simulink model "atrias_system"  (R2015a)
settings: Solver=FixedStepDiscrete  StartTime=0.0  StopTime=inf  FixedStep=sample_time  RelTol=1e-3
undefined symbols (not defined in the file or in its folder): gui_disable_cmd, gui_enable_cmd, gui_estop_cmd, gui_reset_cmd, HIP_CURRENT_LIMIT, HIP_MOTOR_CONSTANT, HIP_MTR_GEAR_RATIO, HIP_MTR_MAX_TORQUE, LEFT_MOTOR_HIP_DIRECTION, LEG1_MOTOR_A_DIRECTION, LEG1_MOTOR_B_DIRECTION, LEG2_MOTOR_A_DIRECTION, LEG2_MOTOR_B_DIRECTION, LEG_CURRENT_LIMIT, LEG_MOTOR_CONSTANT, LEG_MTR_GEAR_RATIO, LEG_MTR_MAX_TORQUE, MEDULLA_ADC_MAX_VOLTS, MEDULLA_ADC_OFFSET_COUNTS, MEDULLA_STATE_ERROR, MEDULLA_STATE_HALT, MEDULLA_STATE_IDLE, MEDULLA_STATE_RESET, MEDULLA_STATE_RUN, MOTOR_POSITION_LIMITS_LOWER, MOTOR_POSITION_LIMITS_UPPER, MTR_HIP_MAX_CURRENT, MTR_MAX_CONT_CURRENT, MTR_MAX_COUNT, MTR_MAX_CURRENT, RIGHT_MOTOR_HIP_DIRECTION
libraries: xpcethercatlib x188, simulink x36, slrtlib x2
(part 1 of 3)
settings Model: SimulationMode=external  CovSFcnEnable=off  Creator=wmartin  LastModifiedBy=robots
settings SolverCC: EnableConcurrentExecution=on
settings DataIOCC: MaxDataPoints=1000000000  SaveFormat=StructureWithTime  SaveOutput=off  SaveTime=off
settings OptimizationCC: BlockReduction=off  OptimizeBlockIOStorage=off  BufferReuse=off  GlobalBufferReuse=off  ExpressionFolding=off  ExpressionDepthLimit=2147483647  LocalBlockOutputs=off  SimCompilerOptimization=on
settings DebuggingCC: UnderspecifiedInitializationDetection=Classic  MergeDetectMultiDrivingBlocksExec=none  SolverPrmCheckMsg=warning  StateNameClashWarn=warning
settings HardwareCC: ProdIntDivRoundTo=Zero  ProdEndianess=LittleEndian  ProdLongLongMode=on  ProdHWDeviceType=Generic->32-bit x86 compatible
settings ModelReferenceCC: EnableParallelModelReferenceBuilds=on  ModelReferenceNumInstancesAllowed=Single  ModelReferenceMinAlgLoopOccurrences=on
settings RTWCC: SystemTargetFile=slrt.tlc  TemplateMakefile=slrt_default_tmf  Description=Simulink Real-Time  RTWVerbose=off  RTWCompilerOptimization=on
settings CodeAppCC: MaxIdLength=256
settings SimulinkRealTimeCC: GeneratePreprocessorConditionals=Disable all  RL32LogBufSizeModifier=100000000

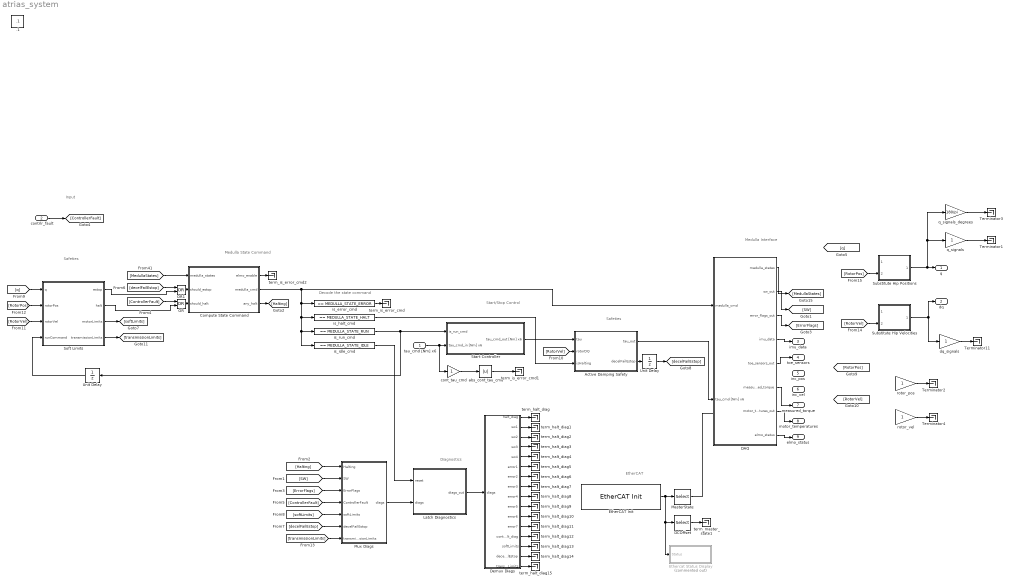
== system atrias_system ==
  note: Decode the state command
  note: Medulla Interface
  note: Medulla State Command
  note: Diagnostics
  note: EtherCAT
  note: Start/Stop Control
  note: Input
  note: Safeties
  note: Safeties
  tau_cmd [Nm] x6 : Inport
  contrlr_fault : Inport  Port=2  OutDataTypeStr=boolean
  Active Damping Safety : MATLAB Function  TreatAsAtomicUnit=on
  Compute State Command : MATLAB Function  TreatAsAtomicUnit=on
  DAQ : Subsystem
  DCOffset : Selector  InputPortWidth=6  Indices=[4]
  Demux Diags : MATLAB Function  TreatAsAtomicUnit=on
  EtherCAT Init : xpcethercatlib/EtherCAT Init   Priority=0  config_file=7medullas4elmos_eni.xml  device_id=0  pci_bus=2  pci_slot=0  enaDebug=off  enaDC=on  errLink=off  masterDbg=off  stateChgDbg=off  baseClock=off  masterCfg=off  logFile='E:\dbglog.txt'  sample_time=0.001000
  Ethercat Status Display : Subsystem  Commented=on
  Latch Diagnostics : MATLAB Function  TreatAsAtomicUnit=on
  MasterState : Selector  InputPortWidth=6  Indices=[2]
  Mux Diags : MATLAB Function  TreatAsAtomicUnit=on
  OR : Logic  Operator=OR  AllPortsSameDT=off  OutDataTypeStr=boolean
  OR1 : Logic  Operator=OR  AllPortsSameDT=off  OutDataTypeStr=boolean
  Soft Limits : MATLAB Function  TreatAsAtomicUnit=on
  Start Controller : Subsystem
  Substitute Hip Positions : Subsystem
  Substitute Hip Velocities : Subsystem
  Terminator{1..4,11} (5 alike) : Terminator
  Unit Delay : UnitDelay  SampleTime=-1
  "Unit Delay " : UnitDelay  SampleTime=-1
  abs_cont_tau_cmd : Abs
  cont_tau_cmd : Gain
  dq_signals : Gain
  is_error_cmd : simulink/Logic and Bit Operations/Compare To Constant  relop===  const=MEDULLA_STATE_ERROR  OutDataTypeStr=boolean
  is_halt_cmd : simulink/Logic and Bit Operations/Compare To Constant  relop===  const=MEDULLA_STATE_HALT  OutDataTypeStr=boolean
  is_idle_cmd : simulink/Logic and Bit Operations/Compare To Constant  relop===  const=MEDULLA_STATE_IDLE  OutDataTypeStr=boolean
  is_run_cmd : simulink/Logic and Bit Operations/Compare To Constant  relop===  const=MEDULLA_STATE_RUN  OutDataTypeStr=boolean
  q_signals : Gain
  q_signals_degrees : Gain  Gain=180/pi
  rotor_pos : Gain
  rotor_vel : Gain
  term_halt_diag{,1..15} (16 alike) : Terminator
  term_is_error_cmd : Terminator
  term_is_error_cmd1 : Terminator
  term_is_error_cmd2 : Terminator
  term_master_state1 : Terminator
  q : Outport
  dq : Outport  Port=2
  imu_data : Outport  Port=3
  toe_sensors : Outport  Port=4
  inc_pos : Outport  Port=5
  inc_vel : Outport  Port=6
  measured_torque : Outport  Port=7
  motor_temperatures : Outport  Port=8
  elmo_status : Outport  Port=9
  .1 : Constant  IOType=siggen  Value=.1
  wires:
  MasterState/1 -> ?
  [MedullaStates] -> Compute State Command/1(medulla_states)
  Compute State Command/3(any_halt) -> [Halting]
  Latch Diagnostics/1(diags_out) -> Demux Diags/1(diags)
  is_halt_cmd/1 -> Active Damping Safety/3(isHalting)
  is_error_cmd/1 -> term_is_error_cmd/1
  tau_cmd [Nm] x6/1 -> cont_tau_cmd/1, Start Controller/2(tau_cmd_in [Nm] x6)
  Start Controller/1(tau_cmd_out [Nm] x6) -> Active Damping Safety/1(tau)
  is_idle_cmd/1 -> Latch Diagnostics/1(reset)
  DAQ/2(sw_out) -> [SW]
  Mux Diags/1(diags) -> Latch Diagnostics/2(diags)
  [Halting] -> Mux Diags/1(Halting)
  [SW] -> Mux Diags/2(SW)
  Demux Diags/2(sw1) -> term_halt_diag1/1
  Demux Diags/5(sw4) -> term_halt_diag4/1
  Demux Diags/4(sw3) -> term_halt_diag3/1
  Demux Diags/3(sw2) -> term_halt_diag2/1
  DAQ/3(error_flags_out) -> [ErrorFlags]
  [ErrorFlags] -> Mux Diags/3(ErrorFlags)
  Demux Diags/1(halt_diag) -> term_halt_diag/1
  Demux Diags/12(error7) -> term_halt_diag11/1
  Demux Diags/11(error6) -> term_halt_diag10/1
  Demux Diags/10(error5) -> term_halt_diag9/1
  Demux Diags/9(error4) -> term_halt_diag8/1
  Demux Diags/8(error3) -> term_halt_diag7/1
  Demux Diags/7(error2) -> term_halt_diag6/1
  Demux Diags/6(error1) -> term_halt_diag5/1
  abs_cont_tau_cmd/1 -> term_is_error_cmd1/1
  DAQ/4(imu_data) -> imu_data/1
  [ControllerFault] -> Mux Diags/4(ControllerFault)
  Demux Diags/13(contrlr_fault_diag) -> term_halt_diag12/1
  [RotorPos] -> Soft Limits/2(rotorPos)
  [RotorVel] -> Soft Limits/3(rotorVel)
  EtherCAT Init/1 -> DCOffset/1, Ethercat Status Display/1(Status), MasterState/1
  cont_tau_cmd/1 -> abs_cont_tau_cmd/1
  DAQ/5(toe_sensors_out) -> toe_sensors/1
  contrlr_fault/1 -> [ControllerFault]
  [softLimits] -> Mux Diags/5(softLimits)
  Demux Diags/14(softLimits) -> term_halt_diag13/1
  Soft Limits/3(motorLimits) -> [softLimits]
  is_run_cmd/1 -> Unit Delay/1, Start Controller/1(is_run_cmd)
  Active Damping Safety/1(tau_out) -> DAQ/2(tau_cmd [Nm] x6)
  [RotorVel] -> Active Damping Safety/2(rotorDQ)
  DCOffset/1 -> term_master_state1/1
  [q] -> Soft Limits/1(q)
  [decelFailEstop] -> Mux Diags/6(decelFailEstop)
  Demux Diags/15(decelFailEstop) -> term_halt_diag14/1
  DAQ/1(medulla_states) -> [MedullaStates]
  Active Damping Safety/2(decelFailEstop) -> "Unit Delay "/1
  "Unit Delay "/1 -> [decelFailEstop]
  DAQ/6(measured_torque) -> measured_torque/1
  ? -> rotor_vel/1, [RotorVel], inc_vel/1
  [ControllerFault] -> OR/1
  Soft Limits/2(halt) -> OR/2
  OR/1 -> Compute State Command/3(should_halt)
  Unit Delay/1 -> Soft Limits/4(runCommand)
  [decelFailEstop] -> OR1/1
  OR1/1 -> Compute State Command/2(should_estop)
  Soft Limits/1(estop) -> OR1/2
  Soft Limits/4(transmissionLimits) -> [transmissionLimits]
  [transmissionLimits] -> Mux Diags/7(transmissionLimits)
  Demux Diags/16(transmissionLimits) -> term_halt_diag15/1
  DAQ/7(motor_temperatures_out) -> motor_temperatures/1
  [RotorVel] -> Substitute Hip Velocities/2(Incremental)
  ? -> Substitute Hip Positions/1(Absolute), [q]
  [RotorPos] -> Substitute Hip Positions/2(Incremental)
  q_signals/1 -> Terminator1/1
  q_signals_degrees/1 -> Terminator3/1
  dq_signals/1 -> Terminator11/1
  ? -> rotor_pos/1, [RotorPos], inc_pos/1
  rotor_pos/1 -> Terminator2/1
  rotor_vel/1 -> Terminator4/1
  Substitute Hip Positions/1(Substituted) -> q_signals_degrees/1, q_signals/1, q/1
  ? -> Substitute Hip Velocities/1(Absolute)
  Substitute Hip Velocities/1(Substituted) -> dq_signals/1, dq/1
  Compute State Command/2(medulla_cmd) -> is_idle_cmd/1, is_run_cmd/1, is_halt_cmd/1, is_error_cmd/1, DAQ/1(medulla_cmd)
  Compute State Command/1(elmo_enable) -> term_is_error_cmd2/1
  DAQ/8(elmo_status) -> elmo_status/1

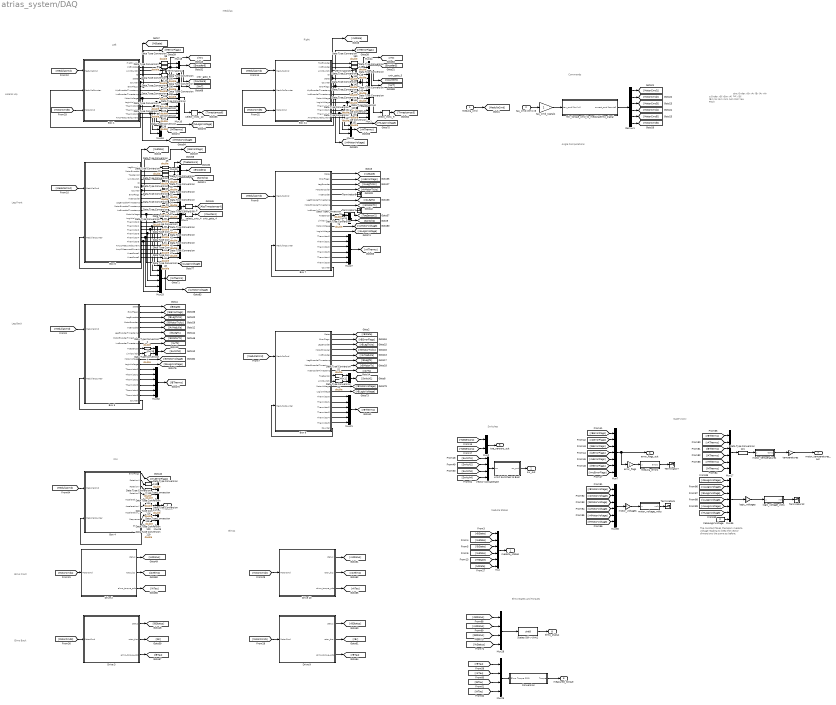
== system atrias_system/DAQ ==
  note: The constant fakes the boom medulla
      | voltage reading to keep the vector
      | dimensions the same as before.
  note: Left
  note: Right
  note: Lateral Hip
  note: Leg Back
  note: Leg Front
  note: Medullas
  note: Angle Computations
  note: Commands
  note: Switches
  note: Supervisory
  note: q Order:
      |
      | rBl
      | rBm
      | rAl
      | rAm
      |
      | lBl
      | lBm
      | lAl
      | lAm
      |
      | rHm
      | lHm
      |
      | Roll
      | Yaw
      | Pitch
  note: Medulla States
  note: IMU
  note: Elmos
  note: Elmo Front
  note: Elmo Back
  note: Elmo States and Torques
  note: qinc Order:
      |
      | rBr
      | rAr
      | lBr
      | lAr
      |
      | rHr
      | lHr
  medulla_cmd : Inport
  tau_cmd [Nm] x6 : Inport  Port=2  OutDataTypeStr=double  PortDimensions=6  SampleTime=0
  Box 1 : Subsystem
  Box 11 : Subsystem
  Box 4 : Subsystem
  Box 5 : Subsystem
  Box 6 : Subsystem
  Box 7 : Subsystem
  Box 8 : Subsystem
  Conversion : Subsystem
  Data Type Conversion{2,4,25..48,51..52,75..76,97..121,138..147,149..151} (68 alike) : DataTypeConversion  OutDataTypeStr=double
  Demux1 : Demux  Outputs=6
  Drive 10 : Subsystem
  Drive 2 : Subsystem
  Drive 3 : Subsystem
  Drive 9 : Subsystem
  FakeLogicVoltage : Constant  Value=0  OutDataTypeStr=uint16
  Limit Switches to Bool : MATLAB Function  TreatAsAtomicUnit=on
  Mux{,17,21,27,32..33,36} (7 alike) : Mux  Inputs=6
  Mux1 : Mux  Inputs=12
  Mux10 : Mux  Inputs=12
  Mux{2,11..14,18,20,24} (8 alike) : Mux  Inputs=2
  Mux25 : Mux
  Mux26 : Mux  Inputs=9
  Mux28 : Mux
  Mux31 : Mux  Inputs=3
  Mux34 : Mux  Inputs=3
  Mux35 : Mux  Inputs=7
  Mux4 : Mux  Inputs=20
  Mux7 : Mux  Inputs=7
  States Dbl->Uint1 : DataTypeConversion  OutDataTypeStr=uint8
  Terminator{1,6..7,9,12,24..25} (7 alike) : Terminator
  Vector Concatenate : Concatenate  NumInputs=4
  error_flags : Gain  OutDataTypeStr=double
  logic_voltage_volts : MATLAB Function  TreatAsAtomicUnit=on
  logic_voltages : Gain  OutDataTypeStr=double
  medulla_errors : MATLAB Function  TreatAsAtomicUnit=on
  motor_temperatures : MATLAB Function  TreatAsAtomicUnit=on
  motor_voltage_volts : MATLAB Function  TreatAsAtomicUnit=on
  motor_voltages : Gain  OutDataTypeStr=double
  mtr_torque_cmd_to_medulla/elmo_signal : Subsystem
  select_cntr_4 : Selector  InputPortWidth=20  Indices=3
  select_incts_10 : Selector  InputPortWidth=12  Indices=[6]
  select_incts_6 : Selector  InputPortWidth=20  Indices=[6 7]
  select_incts_9 : Selector  InputPortWidth=12  Indices=[6]
  tau_cmd_signals : Gain
  temperatures : Gain
  medulla_states : Outport  OutDataTypeStr=uint8
  sw_out : Outport  Port=2
  error_flags_out : Outport  Port=3  OutDataTypeStr=uint8
  imu_data : Outport  Port=4
  toe_sensors_out : Outport  Port=5
  measured_torque : Outport  Port=6
  motor_temperatures_out : Outport  Port=7
  elmo_status : Outport  Port=8
  wires:
  Data Type Conversion98/1 -> Mux18/1
  Data Type Conversion97/1 -> [lHr], Mux18/2
  Data Type Conversion110/1 -> Mux10/1
  Data Type Conversion105/1 -> Mux10/2
  Data Type Conversion107/1 -> [Counter6], Mux10/3
  Data Type Conversion106/1 -> Mux10/4
  Data Type Conversion109/1 -> Mux10/5
  Data Type Conversion101/1 -> Mux10/7
  Data Type Conversion103/1 -> Mux10/8
  Data Type Conversion102/1 -> Mux10/9
  Data Type Conversion100/1 -> Mux10/10
  Data Type Conversion99/1 -> Mux10/11
  mtr_torque_cmd_to_medulla/elmo_signal/1(current_cmd [counts]) -> Demux1/1
  Data Type Conversion48/1 -> Mux4/20
  Data Type Conversion47/1 -> Mux4/19
  Data Type Conversion46/1 -> Mux4/18
  Data Type Conversion45/1 -> Mux4/17
  Data Type Conversion44/1 -> Mux4/16
  Data Type Conversion43/1 -> Mux4/15
  Data Type Conversion42/1 -> Mux4/14
  Data Type Conversion41/1 -> Mux4/13
  Data Type Conversion40/1 -> Mux4/12
  Data Type Conversion39/1 -> Mux4/11
  Data Type Conversion38/1 -> Mux4/10
  Data Type Conversion37/1 -> Mux4/9
  Data Type Conversion36/1 -> Mux4/8
  Data Type Conversion35/1 -> Mux4/7
  Data Type Conversion34/1 -> Mux4/6
  Data Type Conversion33/1 -> Mux4/5
  Data Type Conversion32/1 -> Mux4/4
  Data Type Conversion31/1 -> Mux4/3
  Data Type Conversion30/1 -> Mux4/2
  Data Type Conversion29/1 -> Mux4/1
  Data Type Conversion27/1 -> Mux14/1, [ToeSensor4]
  Data Type Conversion26/1 -> Mux20/2
  Data Type Conversion25/1 -> Mux20/1
  Data Type Conversion2/1 -> Mux13/1
  tau_cmd [Nm] x6/1 -> tau_cmd_signals/1
  Data Type Conversion138/1 -> Mux10/12
  Data Type Conversion75/1 -> Mux11/1, [ToeSensor2]
  Data Type Conversion51/1 -> Mux12/1
  Demux1/1 -> [MotorCmd1]
  Demux1/2 -> [MotorCmd2]
  Demux1/3 -> [MotorCmd3]
  Demux1/4 -> [MotorCmd4]
  Demux1/5 -> [MotorCmd5]
  Demux1/6 -> [MotorCmd6]
  Mux4/1 -> select_incts_6/1, select_cntr_4/1
  Mux18/1 -> [Encoder6]
  Mux20/1 -> [Encoder4]
  Data Type Conversion150/1 -> Mux24/1
  Data Type Conversion149/1 -> [rHr], Mux24/2
  Data Type Conversion146/1 -> Mux1/1
  Data Type Conversion141/1 -> Mux1/2
  Data Type Conversion143/1 -> [Counter5], Mux1/3
  Data Type Conversion142/1 -> Mux1/4
  Data Type Conversion145/1 -> Mux1/5
  Data Type Conversion144/1 -> [rHrT], Mux1/6
  Data Type Conversion111/1 -> Mux1/7
  Data Type Conversion140/1 -> Mux1/8
  Data Type Conversion139/1 -> Mux1/9
  Data Type Conversion104/1 -> Mux1/10
  Data Type Conversion151/1 -> Mux1/11
  Data Type Conversion147/1 -> Mux1/12
  Mux24/1 -> [Encoder5]
  tau_cmd_signals/1 -> mtr_torque_cmd_to_medulla/elmo_signal/1(tau_cmd [Nm] x6)
  motor_voltage_volts/1(volt) -> Terminator6/1
  medulla_errors/1(errors) -> Terminator7/1
  logic_voltage_volts/1(volt) -> Terminator12/1
  medulla_cmd/1 -> [MedullaCmd]
  [Switch1] -> Vector Concatenate/1
  [Switch2] -> Vector Concatenate/2
  [Switch3] -> Vector Concatenate/3
  [Switch4] -> Vector Concatenate/4
  Vector Concatenate/1 -> Limit Switches to Bool/1(sw)
  Limit Switches to Bool/1(sw_out) -> sw_out/1
  Mux7/1 -> error_flags/1, error_flags_out/1
  select_cntr_4/1 -> [Counter4]
  Box 4/4(RotationZ) -> Data Type Conversion114/1
  Box 4/5(AccelerationX) -> Data Type Conversion115/1
  Box 4/6(AccelerationY) -> Data Type Conversion116/1
  Box 4/7(AccelerationZ) -> Data Type Conversion117/1
  Data Type Conversion112/1 -> Mux26/1
  Data Type Conversion113/1 -> Mux26/2
  Data Type Conversion114/1 -> Mux26/3
  Box 4/1(ErrorFlags) -> [imuErrorFlags]
  Data Type Conversion117/1 -> Mux26/6
  Data Type Conversion116/1 -> Mux26/5
  Data Type Conversion115/1 -> Mux26/4
  Mux26/1 -> imu_data/1
  [MedullaCmd] -> Box 4/1(MedullaCmd)
  select_incts_6/1 -> [AbsTimestamps4]
  [rBStatus] -> Mux28/1
  States Dbl->Uint1/1 -> elmo_status/1
  Mux28/1 -> States Dbl->Uint1/1
  [rAStatus] -> Mux28/2
  [lBStatus] -> Mux28/3
  [lAStatus] -> Mux28/4
  select_incts_9/1 -> [Timestamps5]
  Mux1/1 -> select_incts_9/1
  select_incts_10/1 -> [Timestamps6]
  Mux10/1 -> select_incts_10/1
  Box 1/1(HipEncoder) -> Data Type Conversion98/1
  Box 1/2(IncEncoder) -> Data Type Conversion97/1
  Box 1/4(ID) -> Data Type Conversion110/1
  Box 1/5(State) -> [lHState], Data Type Conversion105/1
  Box 1/7(ErrorFlags) -> [lHErrorFlags], Data Type Conversion106/1
  Box 1/8(HipEncoderTimestamp) -> Data Type Conversion109/1
  Box 1/9(IncEncoderTimestamp) -> Data Type Conversion108/1
  Box 1/10(MotorVoltage) -> [lHMotorVoltage], Data Type Conversion101/1
  Box 1/11(LogicVoltage) -> [lHLogicVoltage], Data Type Conversion103/1
  Box 1/12(Thermistor0) -> Mux34/1, Data Type Conversion102/1
  Box 1/13(Thermistor1) -> Mux34/2, Data Type Conversion100/1
  Box 1/14(Thermistor2) -> Mux34/3, Data Type Conversion99/1
  Box 1/15(AmpMeasuredCurrent) -> Data Type Conversion138/1
  [MedullaCmd] -> Box 1/1(MedullaCmd)
  Box 1/6(Counter) -> Box 1/2(MedullaCounter), Data Type Conversion107/1
  [MotorCmd6] -> Box 1/3(MotorCmd)
  [MedullaCmd] -> Box 11/1(MedullaCmd)
  Box 11/6(Counter) -> Data Type Conversion143/1, Box 11/2(MedullaCounter)
  [MotorCmd5] -> Box 11/3(MotorCmd)
  Box 11/1(HipEncoder) -> Data Type Conversion150/1
  Box 11/2(IncEncoder) -> Data Type Conversion149/1
  Box 11/4(ID) -> Data Type Conversion146/1
  Box 11/5(State) -> [rHState], Data Type Conversion141/1
  Box 11/7(ErrorFlags) -> [rHErrorFlags], Data Type Conversion142/1
  Box 11/8(HipEncoderTimestamp) -> Data Type Conversion145/1
  Box 11/9(IncEncoderTimestamp) -> Data Type Conversion144/1
  Box 11/10(MotorVoltage) -> [rHMotorVoltage], Data Type Conversion111/1
  Box 11/11(LogicVoltage) -> [rHLogicVoltage], Data Type Conversion140/1
  Box 11/12(Thermistor0) -> Mux31/1, Data Type Conversion139/1
  Box 11/13(Thermistor1) -> Mux31/2, Data Type Conversion104/1
  Box 11/14(Thermistor2) -> Mux31/3, Data Type Conversion151/1
  Box 11/15(AmpMeasuredCurrent) -> Data Type Conversion147/1
  Box 5/9(ToeSensor) -> Data Type Conversion2/1
  Box 5/10(LimitSwitch) -> Data Type Conversion4/1
  Box 5/1(State) -> [lBState]
  Box 5/2(ErrorFlags) -> [lBErrorFlags]
  Box 5/11(MotorVoltage) -> [lBMotorVoltage]
  Box 5/12(LogicVoltage) -> [lBLogicVoltage]
  Box 5/13(Thermistor0) -> Mux32/1
  Box 5/14(Thermistor1) -> Mux32/2
  Box 5/15(Thermistor2) -> Mux32/3
  Box 5/16(Thermistor3) -> Mux32/4
  Box 5/17(Thermistor4) -> Mux32/5
  Box 5/18(Thermistor5) -> Mux32/6
  [MedullaCmd] -> Box 5/1(MedullaCmd)
  Box 5/19(Counter) -> Box 5/2(MedullaCounter)
  [MotorCmd3] -> Drive 3/1(MotorCmd)
  Drive 3/1(status) -> [lBStatus]
  [MotorCmd1] -> Drive 9/1(MotorCmd)
  Drive 9/1(status) -> [rBStatus]
  [MotorCmd4] -> Drive 2/1(MotorCmd)
  Drive 2/1(status) -> [lAStatus]
  [ToeSensor4] -> Mux2/2
  [ToeSensor2] -> Mux2/1
  Mux2/1 -> toe_sensors_out/1
  Data Type Conversion76/1 -> Mux11/2
  Mux11/1 -> [Switch2]
  Data Type Conversion52/1 -> Mux12/2
  Mux12/1 -> [Switch1]
  Data Type Conversion4/1 -> Mux13/2
  Mux13/1 -> [Switch3]
  Data Type Conversion28/1 -> Mux14/2
  Mux14/1 -> [Switch4]
  error_flags/1 -> medulla_errors/1(u)
  logic_voltages/1 -> logic_voltage_volts/1(u)
  motor_voltages/1 -> motor_voltage_volts/1(u)
  Drive 3/2(rotor_tics) -> [lBr]
  Drive 9/2(rotor_tics) -> [rBr]
  Drive 9/3(elmo_torque_pdo) -> [rBTau]
  Drive 2/3(elmo_torque_pdo) -> [lATau]
  Drive 3/3(elmo_torque_pdo) -> [lBTau]
  [rBTau] -> Mux25/1
  [rATau] -> Mux25/2
  [lBTau] -> Mux25/3
  [lATau] -> Mux25/4
  Mux25/1 -> Conversion/1(Elmo Torque PDO)
  Conversion/1(Torque) -> measured_torque/1
  Data Type Conversion108/1 -> [lHrT], Mux10/6
  motor_temperatures/1(temp) -> temperatures/1
  temperatures/1 -> motor_temperatures_out/1
  Box 1/3(LimitSwitch) -> Terminator24/1
  Box 11/3(LimitSwitch) -> Terminator25/1
  [MedullaCmd] -> Box 6/1(MedullaCmd)
  Box 6/7(Counter) -> Box 6/2(MedullaCounter), Data Type Conversion31/1
  Box 6/1(LegEncoder) -> Data Type Conversion25/1
  Box 6/2(MotorEncoder) -> Data Type Conversion26/1
  Box 6/3(ToeSensor) -> Data Type Conversion27/1
  Box 6/4(LimitSwitch) -> Data Type Conversion28/1
  Box 6/5(ID) -> Data Type Conversion29/1
  Box 6/6(State) -> [lAState], Data Type Conversion30/1
  Box 6/8(ErrorFlags) -> [lAErrorFlags], Data Type Conversion32/1
  Box 6/9(IncEncoder) -> Data Type Conversion33/1
  Box 6/10(LegEncoderTimestamp) -> Data Type Conversion34/1
  Box 6/11(MotorEncoderTimestamp) -> Data Type Conversion35/1
  Box 6/12(IncEncoderTimestamp) -> Data Type Conversion36/1
  Box 6/13(MotorVoltage) -> [lAMotorVoltage], Data Type Conversion37/1
  Box 6/14(LogicVoltage) -> [lALogicVoltage], Data Type Conversion38/1
  Box 6/15(Thermistor0) -> Mux33/1, Data Type Conversion39/1
  Box 6/16(Thermistor1) -> Mux33/2, Data Type Conversion40/1
  Box 6/17(Thermistor2) -> Mux33/3, Data Type Conversion41/1
  Box 6/18(Thermistor3) -> Mux33/4, Data Type Conversion42/1
  Box 6/19(Thermistor4) -> Mux33/5, Data Type Conversion43/1
  Box 6/20(Thermistor5) -> Mux33/6, Data Type Conversion44/1
  Box 6/21(Amp1MeasuredCurrent) -> Data Type Conversion45/1
  Box 6/22(Amp2MeasuredCurrent) -> Data Type Conversion46/1
  Box 6/23(KneeForce1) -> Data Type Conversion47/1
  Box 6/24(KneeForce2) -> Data Type Conversion48/1
  [MedullaCmd] -> Box 7/1(MedullaCmd)
  Box 7/19(Counter) -> Box 7/2(MedullaCounter)
  Box 7/9(ToeSensor) -> Data Type Conversion75/1
  Box 7/10(LimitSwitch) -> Data Type Conversion76/1
  Box 7/1(State) -> [rAState]
  Box 7/11(MotorVoltage) -> [rAMotorVoltage]
  Box 7/12(LogicVoltage) -> [rALogicVoltage]
  Box 7/13(Thermistor0) -> Mux27/1
  Box 7/14(Thermistor1) -> Mux27/2
  Box 7/15(Thermistor2) -> Mux27/3
  Box 7/16(Thermistor3) -> Mux27/4
  Box 7/17(Thermistor4) -> Mux27/5
  Box 7/18(Thermistor5) -> Mux27/6
  [MedullaCmd] -> Box 8/1(MedullaCmd)
  Box 8/19(Counter) -> Box 8/2(MedullaCounter)
  Box 8/9(ToeSensor) -> Data Type Conversion51/1
  Box 8/10(LimitSwitch) -> Data Type Conversion52/1
  Box 8/1(State) -> [rBState]
  Box 8/2(ErrorFlags) -> [rBErrorFlags]
  Box 8/11(MotorVoltage) -> [rBMotorVoltage]
  Box 8/12(LogicVoltage) -> [rBLogicVoltage]
  Box 8/13(Thermistor0) -> Mux21/1
  Box 8/14(Thermistor1) -> Mux21/2
  Box 8/15(Thermistor2) -> Mux21/3
  Box 8/16(Thermistor3) -> Mux21/4
  Box 8/17(Thermistor4) -> Mux21/5
  Box 8/18(Thermistor5) -> Mux21/6
  [MotorCmd2] -> Drive 10/1(MotorCmd)
  Drive 10/1(status) -> [rAStatus]
  Drive 10/3(elmo_torque_pdo) -> [rATau]
  Box 4/8(Sequence) -> Data Type Conversion118/1
  Data Type Conversion118/1 -> Mux26/7
  Box 4/9(Status) -> Data Type Conversion120/1
  Box 4/2(RotationX) -> Data Type Conversion112/1
  Box 4/3(RotationY) -> Data Type Conversion113/1
  Data Type Conversion119/1 -> Mux26/9
  Data Type Conversion120/1 -> Mux26/8
  Drive 2/2(rotor_tics) -> [lArElmo]
  Drive 10/2(rotor_tics) -> [rArElmo]
  [rAState] -> Mux/2
  [rBState] -> Mux/1
  [lBState] -> Mux/3
  [lAState] -> Mux/4
  [rHState] -> Mux/5
  [lHState] -> Mux/6
  Mux/1 -> medulla_states/1
  Box 7/2(ErrorFlags) -> [rAErrorFlags]
  [rBErrorFlags] -> Mux7/1
  [imuErrorFlags] -> Mux7/7
  [lHErrorFlags] -> Mux7/6
  [rHErrorFlags] -> Mux7/5
  [lAErrorFlags] -> Mux7/4
  [lBErrorFlags] -> Mux7/3
  [rAErrorFlags] -> Mux7/2
  Data Type Conversion121/1 -> motor_temperatures/1(u)
  Mux17/1 -> Data Type Conversion121/1
  Mux21/1 -> [rBTherms]
  Mux27/1 -> [rATherms]
  Mux31/1 -> [rHTherms]
  Mux32/1 -> [lBTherms]
  Mux33/1 -> [lATherms]
  Mux34/1 -> [lHTherms]
  [rBTherms] -> Mux17/1
  [rATherms] -> Mux17/2
  [lBTherms] -> Mux17/3
  [lATherms] -> Mux17/4
  [rHTherms] -> Mux17/5
  [lHTherms] -> Mux17/6
  FakeLogicVoltage/1 -> Mux35/7
  Mux35/1 -> logic_voltages/1
  [rBLogicVoltage] -> Mux35/1
  [lHLogicVoltage] -> Mux35/6
  [rHLogicVoltage] -> Mux35/5
  [lALogicVoltage] -> Mux35/4
  [lBLogicVoltage] -> Mux35/3
  [rALogicVoltage] -> Mux35/2
  [rAMotorVoltage] -> Mux36/2
  [rBMotorVoltage] -> Mux36/1
  [lBMotorVoltage] -> Mux36/3
  [lAMotorVoltage] -> Mux36/4
  [rHMotorVoltage] -> Mux36/5
  [lHMotorVoltage] -> Mux36/6
  Mux36/1 -> motor_voltages/1
  Box 4/10(Counter) -> Box 4/2(MedullaCounter), Data Type Conversion119/1
  Box 8/5(IncEncoder) -> [rArMedulla]
  Box 8/8(IncEncoderTimestamp) -> [rArTs]
  Box 8/3(LegEncoder) -> [rBLegTicks]
  Box 8/4(MotorEncoder) -> [rBMotorTicks]
  Box 8/6(LegEncoderTimestamp) -> [rBLegTs]
  Box 8/7(MotorEncoderTimestamp) -> [rBMotorTs]
  Box 7/5(IncEncoder) -> Terminator9/1
  Box 7/8(IncEncoderTimestamp) -> Terminator1/1
  Box 7/7(MotorEncoderTimestamp) -> [rAMotorTs]
  Box 7/6(LegEncoderTimestamp) -> [rALegTs]
  Box 7/4(MotorEncoder) -> [rAMotorTicks]
  Box 7/3(LegEncoder) -> [rALegTicks]
  Box 5/3(LegEncoder) -> [lBLegTicks]
  Box 5/4(MotorEncoder) -> [lBMotorTicks]
  Box 5/5(IncEncoder) -> [lArMedulla]
  Box 5/6(LegEncoderTimestamp) -> [lBLegTs]
  Box 5/7(MotorEncoderTimestamp) -> [lBMotorTs]
  Box 5/8(IncEncoderTimestamp) -> [lArTs]

== system atrias_system/Ethercat Status Display ==
  Status : Inport
  Constant2 : Constant  Value=0  OutDataTypeStr=Inherit: Inherit via back propagation  SampleTime=-1
  Data Type Conversion{,1..6} (7 alike) : DataTypeConversion
  Demux : Demux  Outputs=6
  Discrete Filter2 : DiscreteFilter  Numerator="[0.001568334083281   0.001568334083281]"  Denominator="[1.000000000000000  -0.996863331833438]"  a0EqualsOne=on
  Mux2 : Mux  Inputs=3
  Mux3 : Mux  Inputs=6
  Scope 2 : slrtlib/Displays and Logging/Scope   scopeno=1  scopetype=Target  autostart=on  viewmode=Graphical rolling  formatstr='%f'  grid=on  ylimits=[0,0]  nosamples=10000  noprepostsamples=0  interleave=1  triggermode=FreeRun  triggersignal=1  trigsignalfromport=off  triggerlevel=0.0  triggerslope=Either  triggerscope=1  triggersample=0  filename=data.dat  mode=Lazy  writesize=512  autorestart=off  dynamicfilemode=off  maxwritefilesize=512*1024^2
  Scope 3 : slrtlib/Displays and Logging/Scope   scopeno=3  scopetype=Target  autostart=on  viewmode=Numerical  formatstr='%15.6f'  grid=on  ylimits=[0,0]  nosamples=100  noprepostsamples=0  interleave=1  triggermode=FreeRun  triggersignal=1  trigsignalfromport=off  triggerlevel=0.0  triggerslope=Either  triggerscope=1  triggersample=0  filename=data.dat  mode=Lazy  writesize=512  autorestart=off  dynamicfilemode=off  maxwritefilesize=512*1024^2
  wires:
  Status/1 -> Demux/1
  Demux/4 -> Discrete Filter2/1, Mux2/1
  Discrete Filter2/1 -> Data Type Conversion/1
  Mux2/1 -> Scope 2/1
  Constant2/1 -> Data Type Conversion4/1
  Data Type Conversion4/1 -> Mux2/3
  Mux3/1 -> Scope 3/1
  Data Type Conversion/1 -> Mux3/4, Mux2/2  "MasterRefToClockDiff"
  Data Type Conversion1/1 -> Mux3/1  "ErrVal"
  Data Type Conversion2/1 -> Mux3/2  "MasterState"
  Data Type Conversion3/1 -> Mux3/3  "DCErrVal"
  Data Type Conversion5/1 -> Mux3/5  "DCInitState"
  Data Type Conversion6/1 -> Mux3/6  "RefClockToSlaveDiff"
  Demux/1 -> Data Type Conversion1/1  "ErrVal"
  Demux/2 -> Data Type Conversion2/1  "MasterState"
  Demux/3 -> Data Type Conversion3/1  "DCErrVal"
  Demux/5 -> Data Type Conversion5/1  "DCInitState"
  Demux/6 -> Data Type Conversion6/1  "RefClockToSlaveDiff"

== system atrias_system/Start Controller ==
  note: For GUI
  note: Input Order:
      |
      | backR
      | frontR
      | latR
      | backL
      | frontL
      | latL
  is_run_cmd : Inport  OutDataTypeStr=boolean  PortDimensions=1
  tau_cmd_in [Nm] x6 : Inport  Port=2
  Current Time : Clock
  Enabled time : Sum  Inputs=-+
  Hold Start Time : Subsystem  TreatAsAtomicUnit=on
  Lateral Motor Saturation : Saturate  UpperLimit=HIP_MTR_MAX_TORQUE  LowerLimit=-HIP_MTR_MAX_TORQUE
      settings: AttributesFormatString=Top: %<UpperLimit>\nBottom: %<LowerLimit>
  NOT : Logic  Operator=NOT  IconShape=distinctive  AllPortsSameDT=off  OutDataTypeStr=boolean
  Ramp Rate (Units/sec) : Gain  Gain=.25
  Sagittal Motor Saturation : Saturate  UpperLimit=LEG_MTR_MAX_TORQUE  LowerLimit=-LEG_MTR_MAX_TORQUE
      settings: AttributesFormatString=Top: %<UpperLimit>\nBottom: %<LowerLimit>
  Scaling Factor : Saturate  UpperLimit=1  LowerLimit=0
  Selector : Selector  InputPortWidth=6  Indices=[1 2 4 5 6 3]
  Selector1 : Selector  InputPortWidth=6  Indices=[1 2 3 4]
  Selector2 : Selector  InputPortWidth=6  Indices=[5 6]
  Separated to Tau : Selector  InputPortWidth=6  Indices=[1 2 6 3 4 5]
  Startup Tau Ramp : Product
  Sum : Sum  Inputs=|-+
  Terminator : Terminator
  Vector Concatenate : Concatenate
  is_start_done_cmp : RelationalOperator  Operator=>  OutDataTypeStr=boolean
  tau_cmd_out [Nm] x6 : Outport  OutDataTypeStr=double  PortDimensions=6
  wires:
  NOT/1 -> Hold Start Time/Enable
  is_run_cmd/1 -> NOT/1
  Current Time/1 -> Enabled time/2, Hold Start Time/1(Time In)
  Hold Start Time/1(Time Out) -> Enabled time/1
  Enabled time/1 -> Ramp Rate (Units/sec)/1
  Ramp Rate (Units/sec)/1 -> Scaling Factor/1, Sum/2
  Scaling Factor/1 -> is_start_done_cmp/2, Startup Tau Ramp/1
  Startup Tau Ramp/1 -> tau_cmd_out [Nm] x6/1
  Selector2/1 -> Lateral Motor Saturation/1  "lateral"
  Selector1/1 -> Sagittal Motor Saturation/1  "sagittal"
  tau_cmd_in [Nm] x6/1 -> Selector/1
  Selector/1 -> Selector1/1, Selector2/1
  Sagittal Motor Saturation/1 -> Vector Concatenate/1
  Lateral Motor Saturation/1 -> Vector Concatenate/2
  Vector Concatenate/1 -> Separated to Tau/1
  Separated to Tau/1 -> Startup Tau Ramp/2
  Sum/1 -> is_start_done_cmp/1
  is_start_done_cmp/1 -> Terminator/1

== system atrias_system/Substitute Hip Positions ==
  Absolute : Inport
  Incremental : Inport  Port=2
  Mux1 : Mux  Inputs=2
  Replace Hips with Incremental : Selector  InputPortWidth=19  Indices=[1 2 3 4 5 6 7 8 18 19 11 12 13]
  Reshape : Reshape
  Substituted : Outport
  wires:
  Incremental/1 -> Mux1/2
  Absolute/1 -> Mux1/1
  Replace Hips with Incremental/1 -> Reshape/1
  Mux1/1 -> Replace Hips with Incremental/1
  Reshape/1 -> Substituted/1

== system atrias_system/Substitute Hip Velocities ==
  Absolute : Inport
  Incremental : Inport  Port=2
  Mux1 : Mux  Inputs=2
  Replace Hips with Incremental : Selector  InputPortWidth=19  Indices=[1 2 3 4 5 6 7 8 18 19 11 12 13]
  Reshape : Reshape
  Substituted : Outport
  wires:
  Reshape/1 -> Substituted/1
  Mux1/1 -> Replace Hips with Incremental/1
  Replace Hips with Incremental/1 -> Reshape/1
  Absolute/1 -> Mux1/1
  Incremental/1 -> Mux1/2

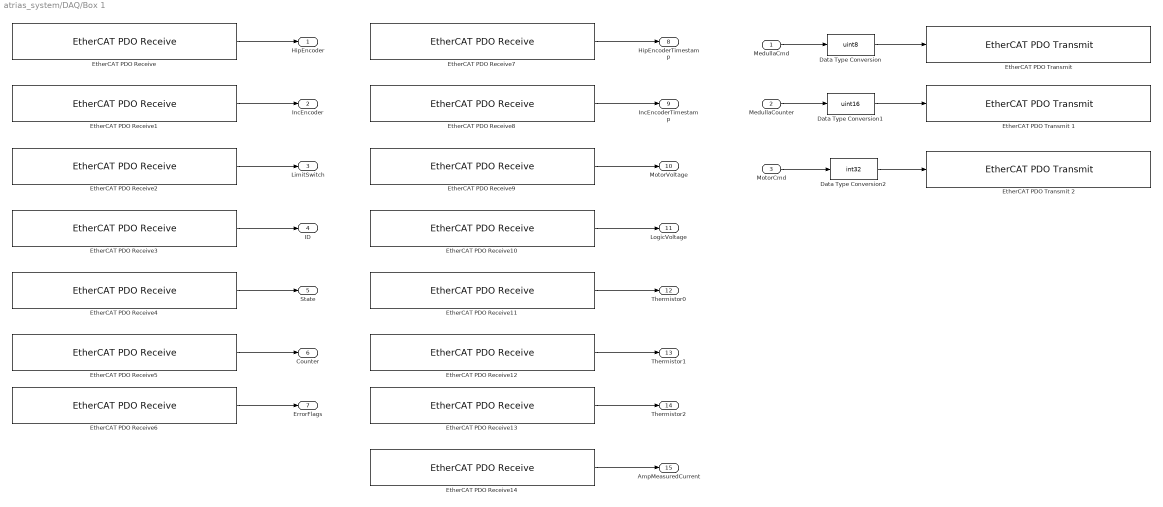
== system atrias_system/DAQ/Box 1 ==
  MedullaCmd : Inport
  MedullaCounter : Inport  Port=2
  MotorCmd : Inport  Port=3
  Data Type Conversion : DataTypeConversion  OutDataTypeStr=uint8
  Data Type Conversion1 : DataTypeConversion  OutDataTypeStr=uint16
  Data Type Conversion2 : DataTypeConversion  OutDataTypeStr=int32
  EtherCAT PDO Receive : xpcethercatlib/EtherCAT PDO Receive  Priority=2  sig_name=Box 1 (ATRIAS 2.1 Hip (Medulla 1.5)).Hip Encoder.Encoder  sig_offset=632  sig_type=uint32  type_size=32  sig_dim=1  device_id=0  sample_time=0.001000
  EtherCAT PDO Receive1 : xpcethercatlib/EtherCAT PDO Receive  Priority=2  sig_name=Box 1 (ATRIAS 2.1 Hip (Medulla 1.5)).Incremental Encoder.Incremental Encoder  sig_offset=776  sig_type=uint16  type_size=16  sig_dim=1  device_id=0  sample_time=0.001000
  EtherCAT PDO Receive10 : xpcethercatlib/EtherCAT PDO Receive  Priority=2  sig_name=Box 1 (ATRIAS 2.1 Hip (Medulla 1.5)).Power.Logic Voltage  sig_offset=696  sig_type=uint16  type_size=16  sig_dim=1  device_id=0  sample_time=0.001000
  EtherCAT PDO Receive11 : xpcethercatlib/EtherCAT PDO Receive  Priority=2  sig_name=Box 1 (ATRIAS 2.1 Hip (Medulla 1.5)).Thermistors.Thermistor 0  sig_offset=712  sig_type=uint16  type_size=16  sig_dim=1  device_id=0  sample_time=0.001000
  EtherCAT PDO Receive12 : xpcethercatlib/EtherCAT PDO Receive  Priority=2  sig_name=Box 1 (ATRIAS 2.1 Hip (Medulla 1.5)).Thermistors.Thermistor 1  sig_offset=728  sig_type=uint16  type_size=16  sig_dim=1  device_id=0  sample_time=0.001000
  EtherCAT PDO Receive13 : xpcethercatlib/EtherCAT PDO Receive  Priority=2  sig_name=Box 1 (ATRIAS 2.1 Hip (Medulla 1.5)).Thermistors.Thermistor 2  sig_offset=744  sig_type=uint16  type_size=16  sig_dim=1  device_id=0  sample_time=0.001000
  EtherCAT PDO Receive14 : xpcethercatlib/EtherCAT PDO Receive  Priority=2  sig_name=Box 1 (ATRIAS 2.1 Hip (Medulla 1.5)).Measured Current.Amp Measured Current  sig_offset=760  sig_type=int16  type_size=16  sig_dim=1  device_id=0  sample_time=0.001000
  EtherCAT PDO Receive2 : xpcethercatlib/EtherCAT PDO Receive  Priority=2  sig_name=Box 1 (ATRIAS 2.1 Hip (Medulla 1.5)).uController Status.Limit Switch  sig_offset=624  sig_type=uint8  type_size=8  sig_dim=1  device_id=0  sample_time=0.001000
  EtherCAT PDO Receive3 : xpcethercatlib/EtherCAT PDO Receive  Priority=2  sig_name=Box 1 (ATRIAS 2.1 Hip (Medulla 1.5)).uController Status.ID  sig_offset=592  sig_type=uint8  type_size=8  sig_dim=1  device_id=0  sample_time=0.001000
  EtherCAT PDO Receive4 : xpcethercatlib/EtherCAT PDO Receive  Priority=2  sig_name=Box 1 (ATRIAS 2.1 Hip (Medulla 1.5)).uController Status.State  sig_offset=600  sig_type=uint8  type_size=8  sig_dim=1  device_id=0  sample_time=0.001000
  EtherCAT PDO Receive5 : xpcethercatlib/EtherCAT PDO Receive  Priority=2  sig_name=Box 1 (ATRIAS 2.1 Hip (Medulla 1.5)).uController Status.Counter  sig_offset=608  sig_type=uint8  type_size=8  sig_dim=1  device_id=0  sample_time=0.001000
  EtherCAT PDO Receive6 : xpcethercatlib/EtherCAT PDO Receive  Priority=2  sig_name=Box 1 (ATRIAS 2.1 Hip (Medulla 1.5)).uController Status.Error Flags  sig_offset=616  sig_type=uint8  type_size=8  sig_dim=1  device_id=0  sample_time=0.001000
  EtherCAT PDO Receive7 : xpcethercatlib/EtherCAT PDO Receive  Priority=2  sig_name=Box 1 (ATRIAS 2.1 Hip (Medulla 1.5)).Hip Encoder.Timestamp  sig_offset=664  sig_type=uint16  type_size=16  sig_dim=1  device_id=0  sample_time=0.001000
  EtherCAT PDO Receive8 : xpcethercatlib/EtherCAT PDO Receive  Priority=2  sig_name=Box 1 (ATRIAS 2.1 Hip (Medulla 1.5)).Incremental Encoder.Incremental Encoder Timestamp  sig_offset=792  sig_type=uint16  type_size=16  sig_dim=1  device_id=0  sample_time=0.001000
  EtherCAT PDO Receive9 : xpcethercatlib/EtherCAT PDO Receive  Priority=2  sig_name=Box 1 (ATRIAS 2.1 Hip (Medulla 1.5)).Power.Motor Voltage  sig_offset=680  sig_type=uint16  type_size=16  sig_dim=1  device_id=0  sample_time=0.001000
  "EtherCAT PDO Transmit " : xpcethercatlib/EtherCAT PDO Transmit   Priority=3  sig_name=Box 1 (ATRIAS 2.1 Hip (Medulla 1.5)).uControllerInput.Command  sig_offset=592  sig_type=uint8  type_size=8  sig_dim=1  device_id=0  sample_time=0.001000
  EtherCAT PDO Transmit 1 : xpcethercatlib/EtherCAT PDO Transmit   Priority=3  sig_name=Box 1 (ATRIAS 2.1 Hip (Medulla 1.5)).uControllerInput.Counter  sig_offset=600  sig_type=uint16  type_size=16  sig_dim=1  device_id=0  sample_time=0.001000
  EtherCAT PDO Transmit 2 : xpcethercatlib/EtherCAT PDO Transmit   Priority=3  sig_name=Box 1 (ATRIAS 2.1 Hip (Medulla 1.5)).uControllerInput.Motor Current  sig_offset=616  sig_type=int32  type_size=32  sig_dim=1  device_id=0  sample_time=0.001000
  HipEncoder : Outport
  IncEncoder : Outport  Port=2
  LimitSwitch : Outport  Port=3
  ID : Outport  Port=4
  State : Outport  Port=5
  Counter : Outport  Port=6
  ErrorFlags : Outport  Port=7
  HipEncoderTimestamp : Outport  Port=8
  IncEncoderTimestamp : Outport  Port=9
  MotorVoltage : Outport  Port=10
  LogicVoltage : Outport  Port=11
  Thermistor0 : Outport  Port=12
  Thermistor1 : Outport  Port=13
  Thermistor2 : Outport  Port=14
  AmpMeasuredCurrent : Outport  Port=15
  wires:
  Data Type Conversion/1 -> "EtherCAT PDO Transmit "/1
  Data Type Conversion1/1 -> EtherCAT PDO Transmit 1/1
  Data Type Conversion2/1 -> EtherCAT PDO Transmit 2/1
  MedullaCmd/1 -> Data Type Conversion/1
  MedullaCounter/1 -> Data Type Conversion1/1
  MotorCmd/1 -> Data Type Conversion2/1
  EtherCAT PDO Receive8/1 -> IncEncoderTimestamp/1
  EtherCAT PDO Receive/1 -> HipEncoder/1
  EtherCAT PDO Receive7/1 -> HipEncoderTimestamp/1
  EtherCAT PDO Receive1/1 -> IncEncoder/1
  EtherCAT PDO Receive5/1 -> Counter/1
  EtherCAT PDO Receive3/1 -> ID/1
  EtherCAT PDO Receive2/1 -> LimitSwitch/1
  EtherCAT PDO Receive4/1 -> State/1
  EtherCAT PDO Receive6/1 -> ErrorFlags/1
  EtherCAT PDO Receive10/1 -> LogicVoltage/1
  EtherCAT PDO Receive9/1 -> MotorVoltage/1
  EtherCAT PDO Receive11/1 -> Thermistor0/1
  EtherCAT PDO Receive12/1 -> Thermistor1/1
  EtherCAT PDO Receive13/1 -> Thermistor2/1
  EtherCAT PDO Receive14/1 -> AmpMeasuredCurrent/1

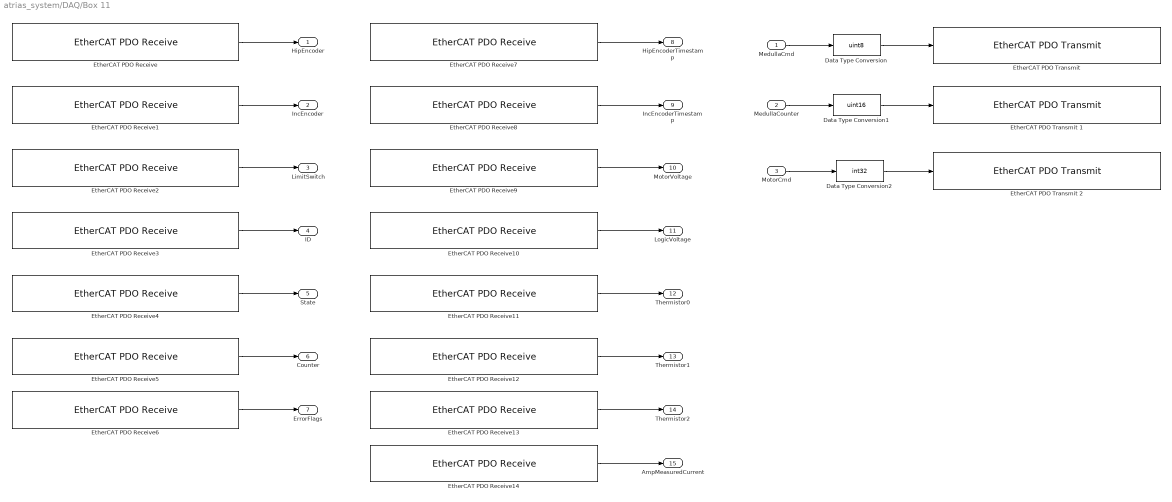
== system atrias_system/DAQ/Box 11 ==
  MedullaCmd : Inport
  MedullaCounter : Inport  Port=2
  MotorCmd : Inport  Port=3
  Data Type Conversion : DataTypeConversion  OutDataTypeStr=uint8
  Data Type Conversion1 : DataTypeConversion  OutDataTypeStr=uint16
  Data Type Conversion2 : DataTypeConversion  OutDataTypeStr=int32
  EtherCAT PDO Receive : xpcethercatlib/EtherCAT PDO Receive  Priority=2  sig_name=Box 11 (ATRIAS 2.1 Hip (Medulla 1.5)).Hip Encoder.Encoder  sig_offset=2640  sig_type=uint32  type_size=32  sig_dim=1  device_id=0  sample_time=0.001000
  EtherCAT PDO Receive1 : xpcethercatlib/EtherCAT PDO Receive  Priority=2  sig_name=Box 11 (ATRIAS 2.1 Hip (Medulla 1.5)).Incremental Encoder.Incremental Encoder  sig_offset=2784  sig_type=uint16  type_size=16  sig_dim=1  device_id=0  sample_time=0.001000
  EtherCAT PDO Receive10 : xpcethercatlib/EtherCAT PDO Receive  Priority=2  sig_name=Box 11 (ATRIAS 2.1 Hip (Medulla 1.5)).Power.Logic Voltage  sig_offset=2704  sig_type=uint16  type_size=16  sig_dim=1  device_id=0  sample_time=0.001000
  EtherCAT PDO Receive11 : xpcethercatlib/EtherCAT PDO Receive  Priority=2  sig_name=Box 11 (ATRIAS 2.1 Hip (Medulla 1.5)).Thermistors.Thermistor 0  sig_offset=2720  sig_type=uint16  type_size=16  sig_dim=1  device_id=0  sample_time=0.001000
  EtherCAT PDO Receive12 : xpcethercatlib/EtherCAT PDO Receive  Priority=2  sig_name=Box 11 (ATRIAS 2.1 Hip (Medulla 1.5)).Thermistors.Thermistor 1  sig_offset=2736  sig_type=uint16  type_size=16  sig_dim=1  device_id=0  sample_time=0.001000
  EtherCAT PDO Receive13 : xpcethercatlib/EtherCAT PDO Receive  Priority=2  sig_name=Box 11 (ATRIAS 2.1 Hip (Medulla 1.5)).Thermistors.Thermistor 2  sig_offset=2752  sig_type=uint16  type_size=16  sig_dim=1  device_id=0  sample_time=0.001000
  EtherCAT PDO Receive14 : xpcethercatlib/EtherCAT PDO Receive  Priority=2  sig_name=Box 11 (ATRIAS 2.1 Hip (Medulla 1.5)).Measured Current.Amp Measured Current  sig_offset=2768  sig_type=int16  type_size=16  sig_dim=1  device_id=0  sample_time=0.001000
  EtherCAT PDO Receive2 : xpcethercatlib/EtherCAT PDO Receive  Priority=2  sig_name=Box 11 (ATRIAS 2.1 Hip (Medulla 1.5)).uController Status.Limit Switch  sig_offset=2632  sig_type=uint8  type_size=8  sig_dim=1  device_id=0  sample_time=0.001000
  EtherCAT PDO Receive3 : xpcethercatlib/EtherCAT PDO Receive  Priority=2  sig_name=Box 11 (ATRIAS 2.1 Hip (Medulla 1.5)).uController Status.ID  sig_offset=2600  sig_type=uint8  type_size=8  sig_dim=1  device_id=0  sample_time=0.001000
  EtherCAT PDO Receive4 : xpcethercatlib/EtherCAT PDO Receive  Priority=2  sig_name=Box 11 (ATRIAS 2.1 Hip (Medulla 1.5)).uController Status.State  sig_offset=2608  sig_type=uint8  type_size=8  sig_dim=1  device_id=0  sample_time=0.001000
  EtherCAT PDO Receive5 : xpcethercatlib/EtherCAT PDO Receive  Priority=2  sig_name=Box 11 (ATRIAS 2.1 Hip (Medulla 1.5)).uController Status.Counter  sig_offset=2616  sig_type=uint8  type_size=8  sig_dim=1  device_id=0  sample_time=0.001000
  EtherCAT PDO Receive6 : xpcethercatlib/EtherCAT PDO Receive  Priority=2  sig_name=Box 11 (ATRIAS 2.1 Hip (Medulla 1.5)).uController Status.Error Flags  sig_offset=2624  sig_type=uint8  type_size=8  sig_dim=1  device_id=0  sample_time=0.001000
  EtherCAT PDO Receive7 : xpcethercatlib/EtherCAT PDO Receive  Priority=2  sig_name=Box 11 (ATRIAS 2.1 Hip (Medulla 1.5)).Hip Encoder.Timestamp  sig_offset=2672  sig_type=uint16  type_size=16  sig_dim=1  device_id=0  sample_time=0.001000
  EtherCAT PDO Receive8 : xpcethercatlib/EtherCAT PDO Receive  Priority=2  sig_name=Box 11 (ATRIAS 2.1 Hip (Medulla 1.5)).Incremental Encoder.Incremental Encoder Timestamp  sig_offset=2800  sig_type=uint16  type_size=16  sig_dim=1  device_id=0  sample_time=0.001000
  EtherCAT PDO Receive9 : xpcethercatlib/EtherCAT PDO Receive  Priority=2  sig_name=Box 11 (ATRIAS 2.1 Hip (Medulla 1.5)).Power.Motor Voltage  sig_offset=2688  sig_type=uint16  type_size=16  sig_dim=1  device_id=0  sample_time=0.001000
  EtherCAT PDO Transmit : xpcethercatlib/EtherCAT PDO Transmit   Priority=3  sig_name=Box 11 (ATRIAS 2.1 Hip (Medulla 1.5)).uControllerInput.Command  sig_offset=2600  sig_type=uint8  type_size=8  sig_dim=1  device_id=0  sample_time=0.001000
  "EtherCAT PDO Transmit 1 " : xpcethercatlib/EtherCAT PDO Transmit   Priority=3  sig_name=Box 11 (ATRIAS 2.1 Hip (Medulla 1.5)).uControllerInput.Counter  sig_offset=2608  sig_type=uint16  type_size=16  sig_dim=1  device_id=0  sample_time=0.001000
  EtherCAT PDO Transmit 2 : xpcethercatlib/EtherCAT PDO Transmit   Priority=3  sig_name=Box 11 (ATRIAS 2.1 Hip (Medulla 1.5)).uControllerInput.Motor Current  sig_offset=2624  sig_type=int32  type_size=32  sig_dim=1  device_id=0  sample_time=0.001000
  HipEncoder : Outport
  IncEncoder : Outport  Port=2
  LimitSwitch : Outport  Port=3
  ID : Outport  Port=4
  State : Outport  Port=5
  Counter : Outport  Port=6
  ErrorFlags : Outport  Port=7
  HipEncoderTimestamp : Outport  Port=8
  IncEncoderTimestamp : Outport  Port=9
  MotorVoltage : Outport  Port=10
  LogicVoltage : Outport  Port=11
  Thermistor0 : Outport  Port=12
  Thermistor1 : Outport  Port=13
  Thermistor2 : Outport  Port=14
  AmpMeasuredCurrent : Outport  Port=15
  wires:
  Data Type Conversion/1 -> EtherCAT PDO Transmit/1
  Data Type Conversion1/1 -> "EtherCAT PDO Transmit 1 "/1
  Data Type Conversion2/1 -> EtherCAT PDO Transmit 2/1
  MedullaCmd/1 -> Data Type Conversion/1
  MedullaCounter/1 -> Data Type Conversion1/1
  MotorCmd/1 -> Data Type Conversion2/1
  EtherCAT PDO Receive8/1 -> IncEncoderTimestamp/1
  EtherCAT PDO Receive/1 -> HipEncoder/1
  EtherCAT PDO Receive7/1 -> HipEncoderTimestamp/1
  EtherCAT PDO Receive1/1 -> IncEncoder/1
  EtherCAT PDO Receive5/1 -> Counter/1
  EtherCAT PDO Receive3/1 -> ID/1
  EtherCAT PDO Receive2/1 -> LimitSwitch/1
  EtherCAT PDO Receive4/1 -> State/1
  EtherCAT PDO Receive6/1 -> ErrorFlags/1
  EtherCAT PDO Receive10/1 -> LogicVoltage/1
  EtherCAT PDO Receive9/1 -> MotorVoltage/1
  EtherCAT PDO Receive11/1 -> Thermistor0/1
  EtherCAT PDO Receive12/1 -> Thermistor1/1
  EtherCAT PDO Receive13/1 -> Thermistor2/1
  EtherCAT PDO Receive14/1 -> AmpMeasuredCurrent/1

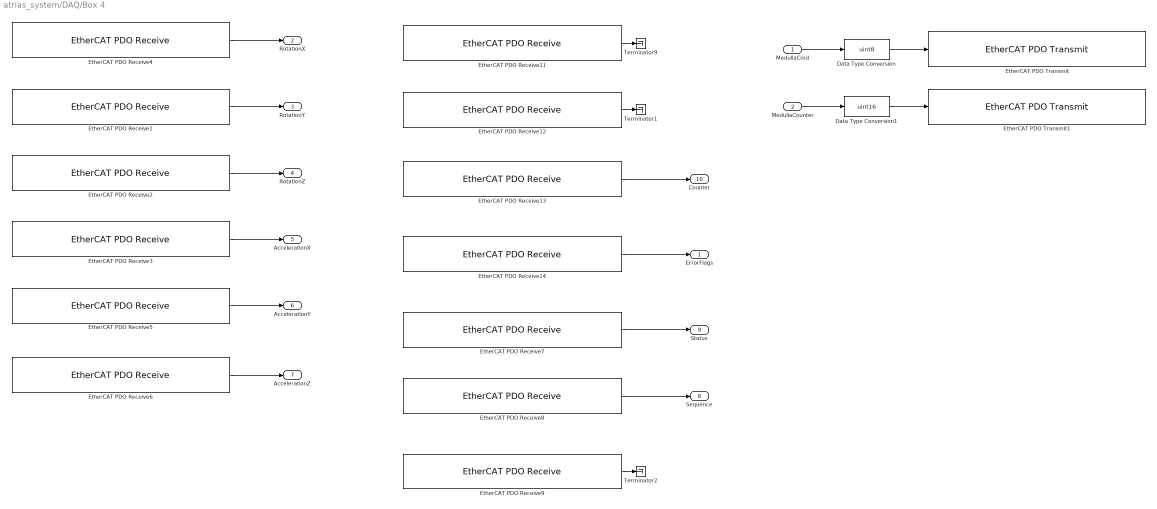
== system atrias_system/DAQ/Box 4 ==
  MedullaCmd : Inport
  MedullaCounter : Inport  Port=2
  Data Type Conversion : DataTypeConversion  OutDataTypeStr=uint8
  Data Type Conversion1 : DataTypeConversion  OutDataTypeStr=uint16
  EtherCAT PDO Receive1 : xpcethercatlib/EtherCAT PDO Receive  Priority=2  sig_name=Box 4 (ATRIAS 2.1 IMU (Medulla 1.5)).Rotation.Y  sig_offset=904  sig_type=single  type_size=32  sig_dim=1  device_id=0  sample_time=0.001000
  EtherCAT PDO Receive11 : xpcethercatlib/EtherCAT PDO Receive  Priority=2  sig_name=Box 4 (ATRIAS 2.1 IMU (Medulla 1.5)).uController Status.ID  sig_offset=840  sig_type=uint8  type_size=8  sig_dim=1  device_id=0  sample_time=0.001000
  EtherCAT PDO Receive12 : xpcethercatlib/EtherCAT PDO Receive  Priority=2  sig_name=Box 4 (ATRIAS 2.1 IMU (Medulla 1.5)).uController Status.State  sig_offset=848  sig_type=uint8  type_size=8  sig_dim=1  device_id=0  sample_time=0.001000
  EtherCAT PDO Receive13 : xpcethercatlib/EtherCAT PDO Receive  Priority=2  sig_name=Box 4 (ATRIAS 2.1 IMU (Medulla 1.5)).uController Status.Counter  sig_offset=856  sig_type=uint8  type_size=8  sig_dim=1  device_id=0  sample_time=0.001000
  EtherCAT PDO Receive14 : xpcethercatlib/EtherCAT PDO Receive  Priority=2  sig_name=Box 4 (ATRIAS 2.1 IMU (Medulla 1.5)).uController Status.Error Flags  sig_offset=864  sig_type=uint8  type_size=8  sig_dim=1  device_id=0  sample_time=0.001000
  EtherCAT PDO Receive2 : xpcethercatlib/EtherCAT PDO Receive  Priority=2  sig_name=Box 4 (ATRIAS 2.1 IMU (Medulla 1.5)).Rotation.Z  sig_offset=936  sig_type=single  type_size=32  sig_dim=1  device_id=0  sample_time=0.001000
  EtherCAT PDO Receive3 : xpcethercatlib/EtherCAT PDO Receive  Priority=2  sig_name=Box 4 (ATRIAS 2.1 IMU (Medulla 1.5)).Acceleration.X  sig_offset=968  sig_type=single  type_size=32  sig_dim=1  device_id=0  sample_time=0.001000
  EtherCAT PDO Receive4 : xpcethercatlib/EtherCAT PDO Receive  Priority=2  sig_name=Box 4 (ATRIAS 2.1 IMU (Medulla 1.5)).Rotation.X  sig_offset=872  sig_type=single  type_size=32  sig_dim=1  device_id=0  sample_time=0.001000
  EtherCAT PDO Receive5 : xpcethercatlib/EtherCAT PDO Receive  Priority=2  sig_name=Box 4 (ATRIAS 2.1 IMU (Medulla 1.5)).Acceleration.Y  sig_offset=1000  sig_type=single  type_size=32  sig_dim=1  device_id=0  sample_time=0.001000
  EtherCAT PDO Receive6 : xpcethercatlib/EtherCAT PDO Receive  Priority=2  sig_name=Box 4 (ATRIAS 2.1 IMU (Medulla 1.5)).Acceleration.Z  sig_offset=1032  sig_type=single  type_size=32  sig_dim=1  device_id=0  sample_time=0.001000
  EtherCAT PDO Receive7 : xpcethercatlib/EtherCAT PDO Receive  Priority=2  sig_name=Box 4 (ATRIAS 2.1 IMU (Medulla 1.5)).Status.Status  sig_offset=1064  sig_type=uint8  type_size=8  sig_dim=1  device_id=0  sample_time=0.001000
  EtherCAT PDO Receive8 : xpcethercatlib/EtherCAT PDO Receive  Priority=2  sig_name=Box 4 (ATRIAS 2.1 IMU (Medulla 1.5)).Status.Sequence  sig_offset=1072  sig_type=uint8  type_size=8  sig_dim=1  device_id=0  sample_time=0.001000
  EtherCAT PDO Receive9 : xpcethercatlib/EtherCAT PDO Receive  Priority=2  sig_name=Box 4 (ATRIAS 2.1 IMU (Medulla 1.5)).Status.Temperature  sig_offset=1080  sig_type=int16  type_size=16  sig_dim=1  device_id=0  sample_time=0.001000
  EtherCAT PDO Transmit : xpcethercatlib/EtherCAT PDO Transmit   Priority=3  sig_name=Box 4 (ATRIAS 2.1 IMU (Medulla 1.5)).uControllerInput.Command  sig_offset=840  sig_type=uint8  type_size=8  sig_dim=1  device_id=0  sample_time=0.001000
  EtherCAT PDO Transmit1 : xpcethercatlib/EtherCAT PDO Transmit   Priority=3  sig_name=Box 4 (ATRIAS 2.1 IMU (Medulla 1.5)).uControllerInput.Counter  sig_offset=848  sig_type=uint16  type_size=16  sig_dim=1  device_id=0  sample_time=0.001000
  Terminator1 : Terminator
  Terminator2 : Terminator
  Terminator9 : Terminator
  ErrorFlags : Outport
  RotationX : Outport  Port=2
  RotationY : Outport  Port=3
  RotationZ : Outport  Port=4
  AccelerationX : Outport  Port=5
  AccelerationY : Outport  Port=6
  AccelerationZ : Outport  Port=7
  Sequence : Outport  Port=8
  Status : Outport  Port=9
  Counter : Outport  Port=10
  wires:
  EtherCAT PDO Receive8/1 -> Sequence/1
  EtherCAT PDO Receive7/1 -> Status/1
  EtherCAT PDO Receive6/1 -> AccelerationZ/1
  EtherCAT PDO Receive5/1 -> AccelerationY/1
  EtherCAT PDO Receive3/1 -> AccelerationX/1
  EtherCAT PDO Receive2/1 -> RotationZ/1
  EtherCAT PDO Receive1/1 -> RotationY/1
  EtherCAT PDO Receive4/1 -> RotationX/1
  MedullaCounter/1 -> Data Type Conversion1/1
  MedullaCmd/1 -> Data Type Conversion/1
  Data Type Conversion1/1 -> EtherCAT PDO Transmit1/1
  Data Type Conversion/1 -> EtherCAT PDO Transmit/1
  EtherCAT PDO Receive13/1 -> Counter/1
  EtherCAT PDO Receive14/1 -> ErrorFlags/1
  EtherCAT PDO Receive11/1 -> Terminator9/1
  EtherCAT PDO Receive12/1 -> Terminator1/1
  EtherCAT PDO Receive9/1 -> Terminator2/1
